simulink model "P4_Hipotenso"  (R2024b)
settings: Solver=ode15s  StartTime=1E-3  StopTime=10  MaxStep=1E-3  RelTol=1e-3
libraries: slpidlib x1
settings Model: Creator=mluser
settings DataIOCC: ReturnWorkspaceOutputs=off  TimeSaveName=t
settings DebuggingCC: AlgebraicLoopMsg=none  ArtificialAlgebraicLoopMsg=none  InheritedTsInSrcMsg=none
settings RTWCC: GPUComputeCapability=3.5

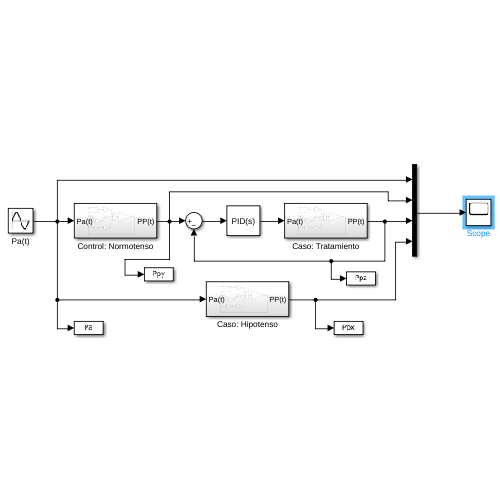
[thumbnail: Simulink's stored preview of the top-level diagram]
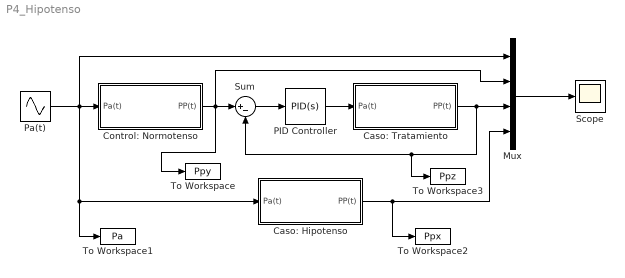
== system P4_Hipotenso ==
  Caso: Hipotenso : Subsystem
  Caso: Tratamiento : Subsystem
  Control: Normotenso : Subsystem
  Mux : Mux
  PID Controller : slpidlib/PID Controller  Controller=PID  Form=Parallel  TimeDomain=Continuous-time  UseExternalTs=off  SampleTime=-1  IntegratorMethod=Forward Euler  FilterMethod=Forward Euler  ControllerParametersSource=internal  P=1E+5  I=4006.6316620614  UseKiTs=off  D=0  UseExternalDerivativeSource=off  N=100  UseFilter=on  TunerSelectOption=Transfer Function Based (PID Tuner App)  InitialConditionSource=internal  InitialConditionForIntegrator=0  InitialConditionForFilter=0  DifferentiatorICPrevScaledInput=0  ExternalReset=none  TrackingMode=off  Kt=1  LimitOutput=off  SatLimitsSource=internal  UpperSaturationLimit=inf  LowerSaturationLimit=-inf  LinearizeAsGain=on  AntiWindupMode=none  Kb=1  LimitIntegrator=off  UpperIntegratorSaturationLimit=inf  LowerIntegratorSaturationLimit=-inf  POutMin=[]  POutMax=[]  IOutMin=[]  IOutMax=[]  DOutMin=[]  DOutMax=[]  NOutMin=[]  NOutMax=[]  SumOutMin=[]  SumOutMax=[]  SaturationOutMin=[]  SaturationOutMax=[]  PParamMin=[]  PParamMax=[]  IParamMin=[]  IParamMax=[]  DParamMin=[]  DParamMax=[]  NParamMin=[]  NParamMax=[]  KbParamMin=[]  KbParamMax=[]  KtParamMin=[]  KtParamMax=[]  KbOutMin=[]  KbOutMax=[]  KtOutMin=[]  KtOutMax=[]  IntegratorOutMin=[]  IntegratorOutMax=[]  FilterOutMin=[]  FilterOutMax=[]  SumI1OutMin=[]  SumI1OutMax=[]  SumI2OutMin=[]  SumI2OutMax=[]  SumI3OutMin=[]  SumI3OutMax=[]  SumI4OutMin=[]  SumI4OutMax=[]  SumDOutMin=[]  SumDOutMax=[]  DifferentiatorOutMin=[]  DifferentiatorOutMax=[]  FilterDiffOutCoefMin=[]  FilterDiffOutCoefMax=[]  ReciprocalOutMin=[]  ReciprocalOutMax=[]  SumDenOutMin=[]  SumDenOutMax=[]  SumNumOutMin=[]  SumNumOutMax=[]  DivideOutMin=[]  DivideOutMax=[]  UdiffTsProdOutMin=[]  UdiffTsProdOutMax=[]  NTsProdOutMin=[]  NTsProdOutMax=[]  UintegralTsProdOutMin=[]  UintegralTsProdOutMax=[]  UngainTsProdOutMin=[]  UngainTsProdOutMax=[]  ClampingZeroOutDataTypeStr=Inherit: Inherit via back propagation  ClampingZeroOutMin=[]  ClampingZeroOutMax=[]  FilterDenConstantOutDataTypeStr=Inherit: Inherit via back propagation  FilterDenConstantOutMin=[]  FilterDenConstantOutMax=[]  PCopyOutDataTypeStr=Inherit: Inherit via back propagation  PCopyOutMin=[]  PCopyOutMax=[]  NCopyOutDataTypeStr=Inherit: Inherit via back propagation  NCopyOutMin=[]  NCopyOutMax=[]  IntegratorContinuousStateAttributes=''  IntegratorStateMustResolveToSignalObject=off  IntegratorRTWStateStorageClass=Auto  FilterContinuousStateAttributes=''  FilterStateMustResolveToSignalObject=off  FilterRTWStateStorageClass=Auto  ParallelPVariant=InternalParameters  IdealPVariant=Disabled  IVariant=InternalParameters  DVariant=InternalParameters  IntegratorVariant=Continuous  SatVariant=Disabled  AWVariant=Passthrough  PCopyVariant=Disabled  TRVariant=Disabled  FdbkBlocksVariant=Forward  IdealPFdbkVariant=Disabled  SatFdbkVariant=Disabled  DerivativeFilterVariant=ContFilter  NVariant=InternalParameters  NCopyVariant=Disabled  FilterICVariant=InternalICsFilter  IntegratorICVariant=InternalICs  ExternalResetVariant=Disabled  TRSumVariant=Passthrough  SumFdbkVariant=Disabled  SumVariant=Sum_PID  TsampFilterVariant=InternalTs  TsampNgainVariant=Passthrough  TsampIntegralVariant=Disabled_SignalSpec  ExternalSaturationOutDataTypeStr=Inherit: Same as second input  DerivativeSourceVariant=ErrorSignal  PreIntVariant=InternalPreInt
  Pa(t) : Sin  Bias=0.8  Frequency=9.42
  Scope : Scope
  Sum : Sum  Inputs=|+-
  To Workspace : ToWorkspace  VariableName=Ppy  SampleTime=-1
  To Workspace1 : ToWorkspace  VariableName=Pa  SampleTime=-1
  To Workspace2 : ToWorkspace  VariableName=Ppx  SampleTime=-1
  To Workspace3 : ToWorkspace  VariableName=Ppz  SampleTime=-1
  wires:
  Pa(t)/1 -> Control: Normotenso/1(Pa(t)), Mux/1, Caso: Hipotenso/1(Pa(t)), To Workspace1/1
  Sum/1 -> PID Controller/1
  Mux/1 -> Scope/1
  Control: Normotenso/1(PP(t)) -> To Workspace/1, Sum/1, Mux/2
  Caso: Hipotenso/1(PP(t)) -> To Workspace2/1, Mux/4
  Caso: Tratamiento/1(PP(t)) -> Sum/2, To Workspace3/1, Mux/3
  PID Controller/1 -> Caso: Tratamiento/1(Pa(t))

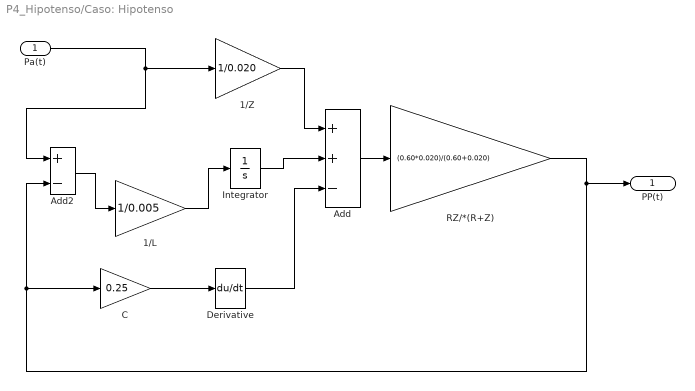
== system P4_Hipotenso/Caso: Hipotenso ==
  Pa(t) : Inport
  1/L : Gain  Gain=1/0.005
  1/Z : Gain  Gain=1/0.020
  Add : Sum  Inputs=++-
  Add2 : Sum  Inputs=+-
  C : Gain  Gain=0.25
  Derivative : Derivative
  Integrator : Integrator
  RZ/*(R+Z) : Gain  Gain=(0.60*0.020)/(0.60+0.020)
  PP(t) : Outport
  wires:
  Derivative/1 -> Add/3
  Add/1 -> RZ/*(R+Z)/1
  RZ/*(R+Z)/1 -> C/1, Add2/2, PP(t)/1
  Pa(t)/1 -> Add2/1, 1/Z/1
  1/L/1 -> Integrator/1
  Integrator/1 -> Add/2
  Add2/1 -> 1/L/1
  1/Z/1 -> Add/1
  C/1 -> Derivative/1

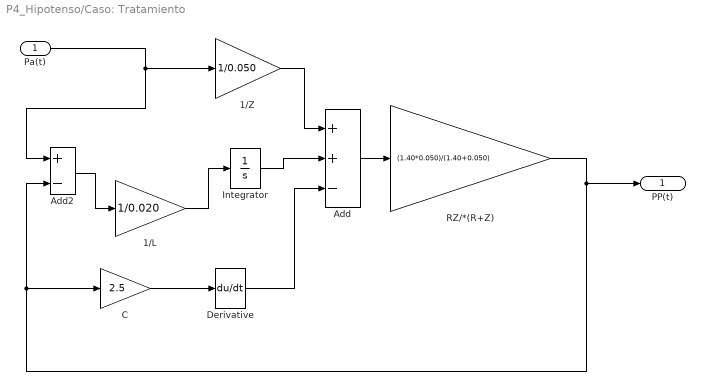
== system P4_Hipotenso/Caso: Tratamiento ==
  Pa(t) : Inport
  1/L : Gain  Gain=1/0.020
  1/Z : Gain  Gain=1/0.050
  Add : Sum  Inputs=++-
  Add2 : Sum  Inputs=+-
  C : Gain  Gain=2.5
  Derivative : Derivative
  Integrator : Integrator
  RZ/*(R+Z) : Gain  Gain=(1.40*0.050)/(1.40+0.050)
  PP(t) : Outport
  wires:
  Derivative/1 -> Add/3
  Add/1 -> RZ/*(R+Z)/1
  RZ/*(R+Z)/1 -> C/1, Add2/2, PP(t)/1
  Pa(t)/1 -> Add2/1, 1/Z/1
  1/L/1 -> Integrator/1
  Integrator/1 -> Add/2
  Add2/1 -> 1/L/1
  1/Z/1 -> Add/1
  C/1 -> Derivative/1

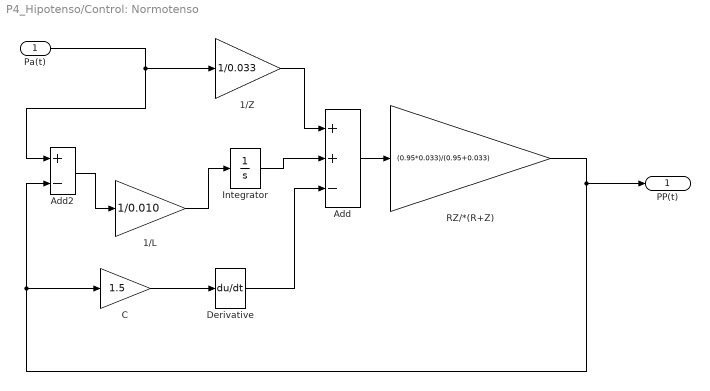
== system P4_Hipotenso/Control: Normotenso ==
  Pa(t) : Inport
  1/L : Gain  Gain=1/0.010
  1/Z : Gain  Gain=1/0.033
  Add : Sum  Inputs=++-
  Add2 : Sum  Inputs=+-
  C : Gain  Gain=1.5
  Derivative : Derivative
  Integrator : Integrator
  RZ/*(R+Z) : Gain  Gain=(0.95*0.033)/(0.95+0.033)
  PP(t) : Outport
  wires:
  Derivative/1 -> Add/3
  Add/1 -> RZ/*(R+Z)/1
  RZ/*(R+Z)/1 -> C/1, Add2/2, PP(t)/1
  Pa(t)/1 -> Add2/1, 1/Z/1
  1/L/1 -> Integrator/1
  Integrator/1 -> Add/2
  Add2/1 -> 1/L/1
  1/Z/1 -> Add/1
  C/1 -> Derivative/1
